simulink model "Attitude_control"  (R2021a)
settings: Solver=VariableStepAuto  StartTime=0.0  StopTime=200  RelTol=1e-3
values from neighbouring files (symbols this model uses):
  D = 9.4e-5*Kt    (= 4.7e-06)    [motor_parameter.m]
  Kt = 0.05    [motor_parameter.m]
  L = 0.001    [motor_parameter.m]
  R = 14.3    [motor_parameter.m]
undefined symbols (not defined in the file or in its folder): b, Is, Km, Q, q_init, Rgyro, Rstr, rw_Inertia, RW_Mmax, rw_SensorToBody, RW_wmax, Ts, unit7, w0, w_dot_init, w_init, wRW_init
libraries: pid_lib x11, simulink_extras x10, sharedtransform x5, simulink x3, aerolibutil x1, sharedTrackingLibrary x1
(part 1 of 2)
settings Model: Creator=sokserey  LastModifiedBy=sokserey

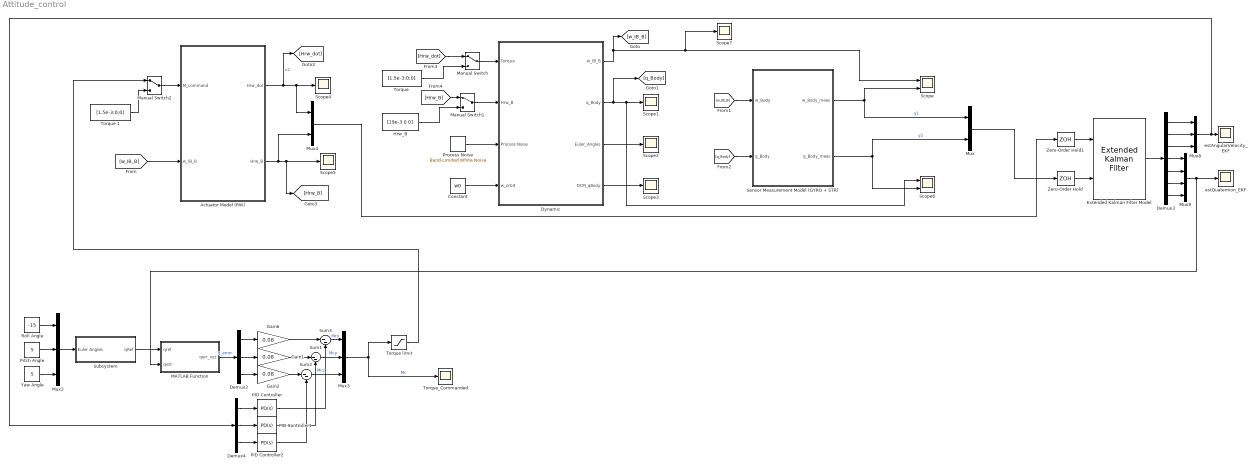
== system Attitude_control ==
  Actuator Model (RW) : Subsystem
  Constant : Constant  Value=w0
  Demux2 : Demux  Outputs=3
  Demux3 : Demux  Outputs=7
  Demux4 : Demux  Outputs=3
  Dynamic : Subsystem
  "Extended Kalman Filter Model " : sharedTrackingLibrary/Extended Kalman Filter  StateTransitionFcn=dynamicFunctions2  HasStateTransitionJacobianFcn=off  HasAdditiveProcessNoise=Additive  ProcessNoise=diag(unit7)*Q  HasTimeVaryingProcessNoise=off  HasStateTransitionFcnExtraArgument=1  InitialState=[w_init; q_init]  InitialStateCovariance=1e-6  MeasurementFcn1=measurementFunction2  HasMeasurementJacobianFcn1=off  HasMeasurementEnablePort1=off  HasAdditiveMeasurementNoise1=Additive  MeasurementNoise1=Rconf4  HasTimeVaryingMeasurementNoise1=off  HasMeasurementFcnExtraArgument1=0  MeasurementFcn2=myMeasurementFcn  HasMeasurementJacobianFcn2=off  HasMeasurementEnablePort2=off  HasAdditiveMeasurementNoise2=Additive  MeasurementNoise2=1  HasTimeVaryingMeasurementNoise2=off  HasMeasurementFcnExtraArgument2=0  MeasurementFcn3=myMeasurementFcn  HasMeasurementJacobianFcn3=off  HasMeasurementEnablePort3=off  HasAdditiveMeasurementNoise3=Additive  MeasurementNoise3=1  HasTimeVaryingMeasurementNoise3=off  HasMeasurementFcnExtraArgument3=0  MeasurementFcn4=myMeasurementFcn  HasMeasurementJacobianFcn4=off  HasMeasurementEnablePort4=off  HasAdditiveMeasurementNoise4=Additive  MeasurementNoise4=1  HasTimeVaryingMeasurementNoise4=off  HasMeasurementFcnExtraArgument4=0  MeasurementFcn5=myMeasurementFcn  HasMeasurementJacobianFcn5=off  HasMeasurementEnablePort5=off  HasAdditiveMeasurementNoise5=Additive  MeasurementNoise5=1  HasTimeVaryingMeasurementNoise5=off  HasMeasurementFcnExtraArgument5=0  EnableMultirate=off  StateTransitionFcnSampleTime=1  MeasurementFcn1SampleTime=1  MeasurementFcn2SampleTime=1  MeasurementFcn3SampleTime=1  MeasurementFcn4SampleTime=1  MeasurementFcn5SampleTime=1  UseCurrentEstimator=on  OutputStateCovariance=off  DataType=double  SampleTime=Ts  NumberOfMeasurements=1
      settings: SourceProductBaseCode=CT,DR,TF,ID,LP,NV,AR,RO,RR,UV,VE
  Gain1 : Gain  Gain=0.08
  Gain2 : Gain  Gain=0.08
  Gain6 : Gain  Gain=0.08
  Hrw_B : Constant  Value=[19e-3 0 0]
  MATLAB Function : MATLAB Function  TreatAsAtomicUnit=on
  Manual Switch : ManualSwitch
  Manual Switch1 : ManualSwitch
  Manual Switch2 : ManualSwitch
  Mux : Mux  Inputs=2
  Mux2 : Mux  Inputs=3
  Mux3 : Mux  Inputs=3
  Mux4 : Mux  Inputs=2
  Mux8 : Mux  Inputs=3
  Mux9 : Mux
  PID Controller : pid_lib/PID Controller  Controller=PD  Form=Parallel  TimeDomain=Continuous-time  UseExternalTs=off  SampleTime=-1  IntegratorMethod=Forward Euler  FilterMethod=Forward Euler  ControllerParametersSource=internal  P=1  I=2  D=2  UseFilter=on  N=100  TunerSelectOption=Transfer Function Based (PID Tuner App)  InitialConditionSource=internal  InitialConditionForIntegrator=0  InitialConditionForFilter=0  DifferentiatorICPrevScaledInput=0  ExternalReset=none  TrackingMode=off  Kt=1  LimitOutput=off  SatLimitsSource=internal  UpperSaturationLimit=inf  LowerSaturationLimit=-inf  LinearizeAsGain=on  AntiWindupMode=none  Kb=1  POutMin=[]  POutMax=[]  IOutMin=[]  IOutMax=[]  DOutMin=[]  DOutMax=[]  NOutMin=[]  NOutMax=[]  SumOutMin=[]  SumOutMax=[]  SaturationOutMin=[]  SaturationOutMax=[]  PParamMin=[]  PParamMax=[]  IParamMin=[]  IParamMax=[]  DParamMin=[]  DParamMax=[]  NParamMin=[]  NParamMax=[]  KbParamMin=[]  KbParamMax=[]  KtParamMin=[]  KtParamMax=[]  KbOutMin=[]  KbOutMax=[]  KtOutMin=[]  KtOutMax=[]  IntegratorOutMin=[]  IntegratorOutMax=[]  FilterOutMin=[]  FilterOutMax=[]  SumI1OutMin=[]  SumI1OutMax=[]  SumI2OutMin=[]  SumI2OutMax=[]  SumI3OutMin=[]  SumI3OutMax=[]  SumI4OutMin=[]  SumI4OutMax=[]  SumDOutMin=[]  SumDOutMax=[]  DifferentiatorOutMin=[]  DifferentiatorOutMax=[]  FilterDiffOutCoefMin=[]  FilterDiffOutCoefMax=[]  ReciprocalOutMin=[]  ReciprocalOutMax=[]  SumDenOutMin=[]  SumDenOutMax=[]  SumNumOutMin=[]  SumNumOutMax=[]  DivideOutMin=[]  DivideOutMax=[]  UdiffTsProdOutMin=[]  UdiffTsProdOutMax=[]  NTsProdOutMin=[]  NTsProdOutMax=[]  UintegralTsProdOutMin=[]  UintegralTsProdOutMax=[]  UngainTsProdOutMin=[]  UngainTsProdOutMax=[]  IntegratorContinuousStateAttributes=''  IntegratorStateMustResolveToSignalObject=off  IntegratorRTWStateStorageClass=Auto  FilterContinuousStateAttributes=''  FilterStateMustResolveToSignalObject=off  FilterRTWStateStorageClass=Auto  ParallelPVariant=InternalParameters  IdealPVariant=Disabled  IVariant=Disabled  DVariant=InternalParameters  IntegratorVariant=Disabled  SatVariant=Disabled  AWVariant=Disabled  PCopyVariant=Disabled  TRVariant=Disabled  FdbkBlocksVariant=Forward  IdealPFdbkVariant=Disabled  SatFdbkVariant=Disabled  DerivativeFilterVariant=ContFilter  NVariant=InternalParameters  NCopyVariant=Disabled  FilterICVariant=InternalICsFilter  IntegratorICVariant=Disabled  ExternalResetVariant=Disabled  TRSumVariant=Passthrough  SumFdbkVariant=Disabled  SumVariant=Sum_PD  TsampFilterVariant=InternalTs  TsampNgainVariant=Passthrough  TsampIntegralVariant=Disabled_SignalSpec  ExternalSaturationOutDataTypeStr=Inherit: Same as second input
  PID Controller1 : pid_lib/PID Controller  Controller=PD  Form=Parallel  TimeDomain=Continuous-time  UseExternalTs=off  SampleTime=-1  IntegratorMethod=Forward Euler  FilterMethod=Forward Euler  ControllerParametersSource=internal  P=1  I=2  D=2  UseFilter=on  N=100  TunerSelectOption=Transfer Function Based (PID Tuner App)  InitialConditionSource=internal  InitialConditionForIntegrator=0  InitialConditionForFilter=0  DifferentiatorICPrevScaledInput=0  ExternalReset=none  TrackingMode=off  Kt=1  LimitOutput=off  SatLimitsSource=internal  UpperSaturationLimit=inf  LowerSaturationLimit=-inf  LinearizeAsGain=on  AntiWindupMode=none  Kb=1  POutMin=[]  POutMax=[]  IOutMin=[]  IOutMax=[]  DOutMin=[]  DOutMax=[]  NOutMin=[]  NOutMax=[]  SumOutMin=[]  SumOutMax=[]  SaturationOutMin=[]  SaturationOutMax=[]  PParamMin=[]  PParamMax=[]  IParamMin=[]  IParamMax=[]  DParamMin=[]  DParamMax=[]  NParamMin=[]  NParamMax=[]  KbParamMin=[]  KbParamMax=[]  KtParamMin=[]  KtParamMax=[]  KbOutMin=[]  KbOutMax=[]  KtOutMin=[]  KtOutMax=[]  IntegratorOutMin=[]  IntegratorOutMax=[]  FilterOutMin=[]  FilterOutMax=[]  SumI1OutMin=[]  SumI1OutMax=[]  SumI2OutMin=[]  SumI2OutMax=[]  SumI3OutMin=[]  SumI3OutMax=[]  SumI4OutMin=[]  SumI4OutMax=[]  SumDOutMin=[]  SumDOutMax=[]  DifferentiatorOutMin=[]  DifferentiatorOutMax=[]  FilterDiffOutCoefMin=[]  FilterDiffOutCoefMax=[]  ReciprocalOutMin=[]  ReciprocalOutMax=[]  SumDenOutMin=[]  SumDenOutMax=[]  SumNumOutMin=[]  SumNumOutMax=[]  DivideOutMin=[]  DivideOutMax=[]  UdiffTsProdOutMin=[]  UdiffTsProdOutMax=[]  NTsProdOutMin=[]  NTsProdOutMax=[]  UintegralTsProdOutMin=[]  UintegralTsProdOutMax=[]  UngainTsProdOutMin=[]  UngainTsProdOutMax=[]  IntegratorContinuousStateAttributes=''  IntegratorStateMustResolveToSignalObject=off  IntegratorRTWStateStorageClass=Auto  FilterContinuousStateAttributes=''  FilterStateMustResolveToSignalObject=off  FilterRTWStateStorageClass=Auto  ParallelPVariant=InternalParameters  IdealPVariant=Disabled  IVariant=Disabled  DVariant=InternalParameters  IntegratorVariant=Disabled  SatVariant=Disabled  AWVariant=Disabled  PCopyVariant=Disabled  TRVariant=Disabled  FdbkBlocksVariant=Forward  IdealPFdbkVariant=Disabled  SatFdbkVariant=Disabled  DerivativeFilterVariant=ContFilter  NVariant=InternalParameters  NCopyVariant=Disabled  FilterICVariant=InternalICsFilter  IntegratorICVariant=Disabled  ExternalResetVariant=Disabled  TRSumVariant=Passthrough  SumFdbkVariant=Disabled  SumVariant=Sum_PD  TsampFilterVariant=InternalTs  TsampNgainVariant=Passthrough  TsampIntegralVariant=Disabled_SignalSpec  ExternalSaturationOutDataTypeStr=Inherit: Same as second input
  PID Controller2 : pid_lib/PID Controller  Controller=PD  Form=Parallel  TimeDomain=Continuous-time  UseExternalTs=off  SampleTime=-1  IntegratorMethod=Forward Euler  FilterMethod=Forward Euler  ControllerParametersSource=internal  P=1  I=2  D=2  UseFilter=on  N=100  TunerSelectOption=Transfer Function Based (PID Tuner App)  InitialConditionSource=internal  InitialConditionForIntegrator=0  InitialConditionForFilter=0  DifferentiatorICPrevScaledInput=0  ExternalReset=none  TrackingMode=off  Kt=1  LimitOutput=off  SatLimitsSource=internal  UpperSaturationLimit=inf  LowerSaturationLimit=-inf  LinearizeAsGain=on  AntiWindupMode=none  Kb=1  POutMin=[]  POutMax=[]  IOutMin=[]  IOutMax=[]  DOutMin=[]  DOutMax=[]  NOutMin=[]  NOutMax=[]  SumOutMin=[]  SumOutMax=[]  SaturationOutMin=[]  SaturationOutMax=[]  PParamMin=[]  PParamMax=[]  IParamMin=[]  IParamMax=[]  DParamMin=[]  DParamMax=[]  NParamMin=[]  NParamMax=[]  KbParamMin=[]  KbParamMax=[]  KtParamMin=[]  KtParamMax=[]  KbOutMin=[]  KbOutMax=[]  KtOutMin=[]  KtOutMax=[]  IntegratorOutMin=[]  IntegratorOutMax=[]  FilterOutMin=[]  FilterOutMax=[]  SumI1OutMin=[]  SumI1OutMax=[]  SumI2OutMin=[]  SumI2OutMax=[]  SumI3OutMin=[]  SumI3OutMax=[]  SumI4OutMin=[]  SumI4OutMax=[]  SumDOutMin=[]  SumDOutMax=[]  DifferentiatorOutMin=[]  DifferentiatorOutMax=[]  FilterDiffOutCoefMin=[]  FilterDiffOutCoefMax=[]  ReciprocalOutMin=[]  ReciprocalOutMax=[]  SumDenOutMin=[]  SumDenOutMax=[]  SumNumOutMin=[]  SumNumOutMax=[]  DivideOutMin=[]  DivideOutMax=[]  UdiffTsProdOutMin=[]  UdiffTsProdOutMax=[]  NTsProdOutMin=[]  NTsProdOutMax=[]  UintegralTsProdOutMin=[]  UintegralTsProdOutMax=[]  UngainTsProdOutMin=[]  UngainTsProdOutMax=[]  IntegratorContinuousStateAttributes=''  IntegratorStateMustResolveToSignalObject=off  IntegratorRTWStateStorageClass=Auto  FilterContinuousStateAttributes=''  FilterStateMustResolveToSignalObject=off  FilterRTWStateStorageClass=Auto  ParallelPVariant=InternalParameters  IdealPVariant=Disabled  IVariant=Disabled  DVariant=InternalParameters  IntegratorVariant=Disabled  SatVariant=Disabled  AWVariant=Disabled  PCopyVariant=Disabled  TRVariant=Disabled  FdbkBlocksVariant=Forward  IdealPFdbkVariant=Disabled  SatFdbkVariant=Disabled  DerivativeFilterVariant=ContFilter  NVariant=InternalParameters  NCopyVariant=Disabled  FilterICVariant=InternalICsFilter  IntegratorICVariant=Disabled  ExternalResetVariant=Disabled  TRSumVariant=Passthrough  SumFdbkVariant=Disabled  SumVariant=Sum_PD  TsampFilterVariant=InternalTs  TsampNgainVariant=Passthrough  TsampIntegralVariant=Disabled_SignalSpec  ExternalSaturationOutDataTypeStr=Inherit: Same as second input
  Pitch Angle : Constant  Value=5
  Process Noise : simulink/Sources/Band-Limited White Noise  Cov=Q*Ts  Ts=Ts  seed=[23341]
  Roll Angle : Constant  Value=-15
  Scope : Scope  NumInputPorts=2
  Scope{1..5,7} (6 alike) : Scope
  Scope6 : Scope  NumInputPorts=2
  Sensor Measurement Model (GYRO + STR) : Subsystem
  Subsystem : Subsystem
  Sum1 : Sum  Inputs=|--
  Sum2 : Sum  Inputs=|--
  Sum3 : Sum  Inputs=|--
  Torque limit : Saturate  UpperLimit=RW_Mmax  LowerLimit=-RW_Mmax
  "Torque " : Constant  Value=[1.5e-3;0;0]
  Torque 1 : Constant  Value=[1.5e-3;0;0]
  Torque_Commanded : Scope
  Yaw Angle : Constant  Value=5
  Zero-Order Hold : ZeroOrderHold  SampleTime=Ts
  Zero-Order Hold1 : ZeroOrderHold  SampleTime=Ts
  estAngularVelocity_EKF : Scope
  "estQuaternion_EKF " : Scope
  wires:
  Process Noise/1 -> Dynamic/3("Process Noise ")
  Constant/1 -> Dynamic/4(w_orbit)
  Dynamic/1(w_IB_B) -> [w_IB_B], Scope7/1, Scope/1
  Dynamic/2(q_Body) -> [q_Body], Scope6/1, Scope1/1
  Dynamic/3(Euler_Angles) -> Scope2/1
  Dynamic/4(DCM_qBody) -> Scope3/1
  Zero-Order Hold1/1 -> "Extended Kalman Filter Model "/1
  Demux3/2 -> Mux8/2
  Demux3/3 -> Mux8/3
  Demux3/6 -> Mux9/3
  Demux3/4 -> Mux9/1
  Mux9/1 -> "estQuaternion_EKF "/1, MATLAB Function/2(qest)
  Demux3/5 -> Mux9/2
  "Extended Kalman Filter Model "/1 -> Demux3/1
  Demux3/1 -> Mux8/1
  Zero-Order Hold/1 -> "Extended Kalman Filter Model "/2
  [w_IB_B] -> Actuator Model (RW)/2(w_IB_B)
  Actuator Model (RW)/1("Hrw_dot ") -> [Hrw_dot], Mux4/1, Scope4/1  "u1"
  Actuator Model (RW)/2(Hrw_B) -> Mux4/2, [Hrw_B], Scope5/1
  [w_IB_B] -> Sensor Measurement Model (GYRO + STR)/1(w_Body)
  Sensor Measurement Model (GYRO + STR)/1(w_Body_meas) -> Mux/1, Scope/2  "y1"
  [q_Body] -> Sensor Measurement Model (GYRO + STR)/2(q_Body)
  Sensor Measurement Model (GYRO + STR)/2(q_Body_meas) -> Mux/2, Scope6/2  "y2"
  Mux/1 -> Zero-Order Hold/1
  Manual Switch/1 -> Dynamic/1(Torque)
  "Torque "/1 -> Manual Switch/2
  Manual Switch1/1 -> Dynamic/2(Hrw_B)
  Hrw_B/1 -> Manual Switch1/2
  [Hrw_dot] -> Manual Switch/1
  [Hrw_B] -> Manual Switch1/1
  Roll Angle/1 -> Mux2/1
  Sum1/1 -> Mux3/2  "Mcy"
  MATLAB Function/1(qerr_xyz) -> Demux2/1  "q_error"
  Demux4/2 -> PID Controller1/1
  PID Controller2/1 -> Sum2/2
  Sum3/1 -> Mux3/1  "Mcx"
  Gain2/1 -> Sum2/1
  PID Controller/1 -> Sum3/2
  PID Controller1/1 -> Sum1/2
  Sum2/1 -> Mux3/3  "Mcz"
  Demux4/1 -> PID Controller/1
  Demux2/2 -> Gain1/1
  Demux2/1 -> Gain6/1
  Gain6/1 -> Sum3/1
  Mux3/1 -> Torque limit/1, Torque_Commanded/1  "Mc"
  Yaw Angle/1 -> Mux2/3
  Subsystem/1(qRef) -> MATLAB Function/1(qref)
  Gain1/1 -> Sum1/1
  Pitch Angle/1 -> Mux2/2
  Mux2/1 -> Subsystem/1(Euler Angles)
  Demux2/3 -> Gain2/1
  Mux8/1 -> Demux4/1, estAngularVelocity_EKF/1
  Demux4/3 -> PID Controller2/1
  Torque limit/1 -> Manual Switch2/1
  Manual Switch2/1 -> Actuator Model (RW)/1("M_command ")
  Torque 1/1 -> Manual Switch2/2
  Demux3/7 -> Mux9/4
  Mux4/1 -> Zero-Order Hold1/1

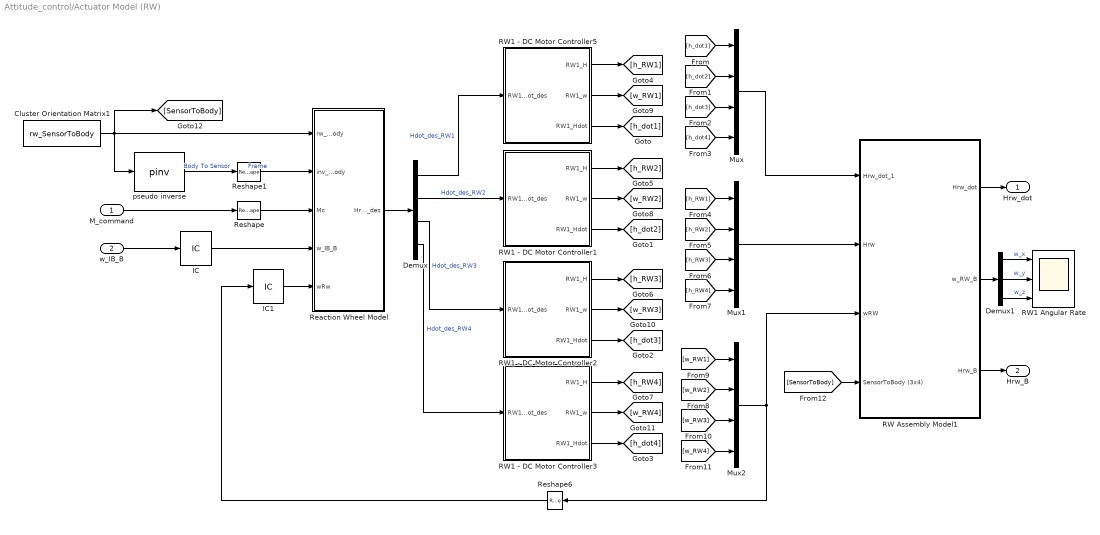
== system Attitude_control/Actuator Model (RW) ==
  "M_command " : Inport
  w_IB_B : Inport  Port=2
  Cluster Orientation Matrix1 : Constant  Value=rw_SensorToBody  VectorParams1D=off  SampleTime=Ts
  Demux : Demux
  Demux1 : Demux  Outputs=3
  IC : InitialCondition  Value=w_init
  IC1 : InitialCondition  Value=wRW_init
  Mux : Mux
  Mux1 : Mux
  Mux2 : Mux
  RW Assembly Model1 : Subsystem
  RW1 - DC Motor Controller1 : Subsystem
  RW1 - DC Motor Controller2 : Subsystem
  RW1 - DC Motor Controller3 : Subsystem
  RW1 - DC Motor Controller5 : Subsystem
  RW1 Angular Rate : Scope  NumInputPorts=3
  Reaction Wheel Model : MATLAB Function  TreatAsAtomicUnit=on
  Reshape : Reshape  OutputDimensionality=Column vector (2-D)
  Reshape1 : Reshape  OutputDimensionality=Customize  OutputDimensions=[4,3]
  Reshape6 : Reshape  OutputDimensionality=Column vector (2-D)
  pseudo inverse : MATLABFcn  MATLABFcn=pinv
  "Hrw_dot " : Outport  VectorParamsAs1DForOutWhenUnconnected=off
  Hrw_B : Outport  Port=2  VectorParamsAs1DForOutWhenUnconnected=off
  wires:
  Demux/1 -> RW1 - DC Motor Controller5/1(RW1_Hdot_des)  "Hdot_des_RW1"
  Demux/2 -> RW1 - DC Motor Controller1/1(RW1_Hdot_des)  "Hdot_des_RW2"
  Demux/3 -> RW1 - DC Motor Controller2/1(RW1_Hdot_des)  "Hdot_des_RW3"
  Demux/4 -> RW1 - DC Motor Controller3/1(RW1_Hdot_des)  "Hdot_des_RW4"
  Demux1/3 -> RW1 Angular Rate/3  "w_z"
  Demux1/1 -> RW1 Angular Rate/1  "w_x"
  Demux1/2 -> RW1 Angular Rate/2  "w_y"
  "M_command "/1 -> Reshape/1
  Reaction Wheel Model/1(Hrw_dot_des) -> Demux/1
  [h_dot1] -> Mux/1
  [h_dot2] -> Mux/2
  [h_dot3] -> Mux/3
  [h_dot4] -> Mux/4
  Mux/1 -> RW Assembly Model1/1(Hrw_dot_1)
  [h_RW1] -> Mux1/1
  [h_RW2] -> Mux1/2
  [h_RW3] -> Mux1/3
  [h_RW4] -> Mux1/4
  Mux1/1 -> RW Assembly Model1/2(Hrw)
  [w_RW2] -> Mux2/2
  [w_RW1] -> Mux2/1
  [w_RW3] -> Mux2/3
  [w_RW4] -> Mux2/4
  pseudo inverse/1 -> Reshape1/1  "Body To Sensor         Frame"
  Reshape/1 -> Reaction Wheel Model/3(Mc)
  Cluster Orientation Matrix1/1 -> pseudo inverse/1, [SensorToBody], Reaction Wheel Model/1(rw_SensorToBody)
  [SensorToBody] -> RW Assembly Model1/4(SensorToBody (3x4))
  RW Assembly Model1/2(w_RW_B) -> Demux1/1
  RW Assembly Model1/1(Hrw_dot) -> "Hrw_dot "/1
  Mux2/1 -> Reshape6/1, RW Assembly Model1/3(wRW)
  Reshape6/1 -> IC1/1
  Reshape1/1 -> Reaction Wheel Model/2(inv_rwSensorToBody)
  w_IB_B/1 -> IC/1
  IC/1 -> Reaction Wheel Model/4(w_IB_B)
  IC1/1 -> Reaction Wheel Model/5(wRw)
  RW1 - DC Motor Controller5/2(RW1_w) -> [w_RW1]
  RW1 - DC Motor Controller5/1(RW1_H) -> [h_RW1]
  RW1 - DC Motor Controller5/3(RW1_Hdot) -> [h_dot1]
  RW1 - DC Motor Controller1/1(RW1_H) -> [h_RW2]
  RW1 - DC Motor Controller1/2(RW1_w) -> [w_RW2]
  RW1 - DC Motor Controller1/3(RW1_Hdot) -> [h_dot2]
  RW1 - DC Motor Controller2/1(RW1_H) -> [h_RW3]
  RW1 - DC Motor Controller2/2(RW1_w) -> [w_RW3]
  RW1 - DC Motor Controller2/3(RW1_Hdot) -> [h_dot3]
  RW1 - DC Motor Controller3/1(RW1_H) -> [h_RW4]
  RW1 - DC Motor Controller3/2(RW1_w) -> [w_RW4]
  RW1 - DC Motor Controller3/3(RW1_Hdot) -> [h_dot4]
  RW Assembly Model1/3(Hrw_B) -> Hrw_B/1

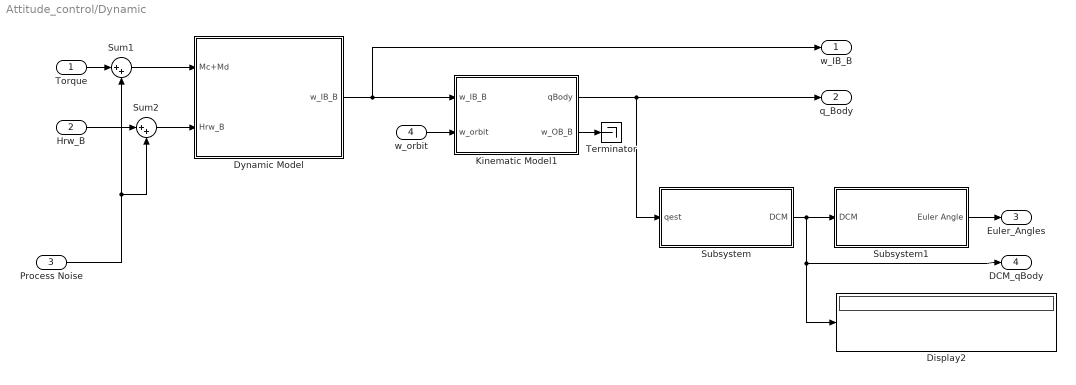
== system Attitude_control/Dynamic ==
  Torque : Inport
  Hrw_B : Inport  Port=2
  "Process Noise " : Inport  Port=3
  w_orbit : Inport  Port=4
  Display2 : Display
  Dynamic Model : Subsystem
  Kinematic Model1 : Subsystem
  Subsystem : Subsystem
  Subsystem1 : Subsystem
  Sum1 : Sum  Inputs=|++
  Sum2 : Sum  Inputs=|++
  Terminator : Terminator
  w_IB_B : Outport  VectorParamsAs1DForOutWhenUnconnected=off
  q_Body : Outport  Port=2  VectorParamsAs1DForOutWhenUnconnected=off
  Euler_Angles : Outport  Port=3  VectorParamsAs1DForOutWhenUnconnected=off
  DCM_qBody : Outport  Port=4  VectorParamsAs1DForOutWhenUnconnected=off
  wires:
  Sum2/1 -> Dynamic Model/2("Hrw_B ")
  Dynamic Model/1(w_IB_B) -> Kinematic Model1/1(w_IB_B), w_IB_B/1
  Hrw_B/1 -> Sum2/1
  Sum1/1 -> Dynamic Model/1(Mc+Md)
  Subsystem1/1(Euler Angle) -> Euler_Angles/1
  Torque/1 -> Sum1/1
  Kinematic Model1/2(w_OB_B) -> Terminator/1
  Kinematic Model1/1(qBody) -> Subsystem/1(qest), q_Body/1
  "Process Noise "/1 -> Sum2/2, Sum1/2
  Subsystem/1("DCM ") -> Display2/1, DCM_qBody/1, Subsystem1/1("DCM ")
  w_orbit/1 -> Kinematic Model1/2(w_orbit)

== system Attitude_control/Sensor Measurement Model (GYRO + STR) ==
  w_Body : Inport
  q_Body : Inport  Port=2
  GYRO Sensor Model : Subsystem
  Normalization Model : Subsystem
  Star Tracker Model : Subsystem
  w_Body_meas : Outport  VectorParamsAs1DForOutWhenUnconnected=off
  q_Body_meas : Outport  Port=2  VectorParamsAs1DForOutWhenUnconnected=off
  wires:
  GYRO Sensor Model/1(w_Body_meas) -> w_Body_meas/1
  w_Body/1 -> GYRO Sensor Model/1(w_Body)
  q_Body/1 -> Star Tracker Model/1(q_Body)
  Normalization Model/1(Normalized_u) -> q_Body_meas/1
  Star Tracker Model/1(q_Body_meas) -> Normalization Model/1(u)

== system Attitude_control/Subsystem ==
  Euler Angles : Inport
  Degrees to Radians1 : simulink_extras/Transformations/Degrees to Radians
  Direction Cosine Matrix to Quaternions : sharedtransform/Direction Cosine Matrix  to Quaternions  aMode=0  action=None  tolerance=eps(2)
      settings: SourceProductBaseCode=AE,PW,DR,MT,UV,VE
  Rotation Angles to Direction Cosine Matrix : sharedtransform/Rotation Angles to Direction Cosine Matrix  rotationOrder=ZYX  aMode=aMode
      settings: SourceProductBaseCode=AE,PW,DR,MT,UV,VE
  Subsystem1 : Subsystem
  qRef : Outport  VectorParamsAs1DForOutWhenUnconnected=off
  wires:
  Euler Angles/1 -> Degrees to Radians1/1
  Degrees to Radians1/1 -> Rotation Angles to Direction Cosine Matrix/1
  Rotation Angles to Direction Cosine Matrix/1 -> Direction Cosine Matrix to Quaternions/1
  Direction Cosine Matrix to Quaternions/1 -> Subsystem1/1(q0,q1,q2,q3)
  Subsystem1/1(q1,q2,q3,q4) -> qRef/1

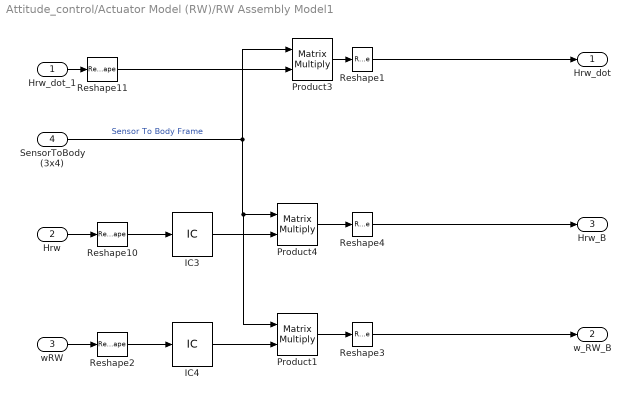
== system Attitude_control/Actuator Model (RW)/RW Assembly Model1 ==
  Hrw_dot_1 : Inport
  Hrw : Inport  Port=2
  wRW : Inport  Port=3
  SensorToBody (3x4) : Inport  Port=4
  IC3 : InitialCondition  Value=[wRW_init(1,1)*rw_Inertia; wRW_init(2,1)*rw_Inertia; wRW_init(3,1)*rw_Inertia;wRW_init(4,1)*rw_Inertia]
  IC4 : InitialCondition  Value=wRW_init
  Product1 : Product  Inputs=**  Multiplication=Matrix(*)  RndMeth=Zero
  Product3 : Product  Inputs=**  Multiplication=Matrix(*)  RndMeth=Zero
  Product4 : Product  Inputs=**  Multiplication=Matrix(*)  RndMeth=Zero
  Reshape{1..4,10..11} (6 alike) : Reshape  OutputDimensionality=Column vector (2-D)
  Hrw_dot : Outport  VectorParamsAs1DForOutWhenUnconnected=off
  w_RW_B : Outport  Port=2  VectorParamsAs1DForOutWhenUnconnected=off
  Hrw_B : Outport  Port=3  VectorParamsAs1DForOutWhenUnconnected=off
  wires:
  SensorToBody (3x4)/1 -> Product3/1, Product1/1, Product4/1  "Sensor To Body Frame"
  Product4/1 -> Reshape4/1
  Reshape1/1 -> Hrw_dot/1
  Reshape4/1 -> Hrw_B/1
  IC3/1 -> Product4/2
  IC4/1 -> Product1/2
  Product1/1 -> Reshape3/1
  Hrw/1 -> Reshape10/1
  Reshape10/1 -> IC3/1
  Reshape2/1 -> IC4/1
  wRW/1 -> Reshape2/1
  Reshape3/1 -> w_RW_B/1
  Reshape11/1 -> Product3/2
  Hrw_dot_1/1 -> Reshape11/1
  Product3/1 -> Reshape1/1

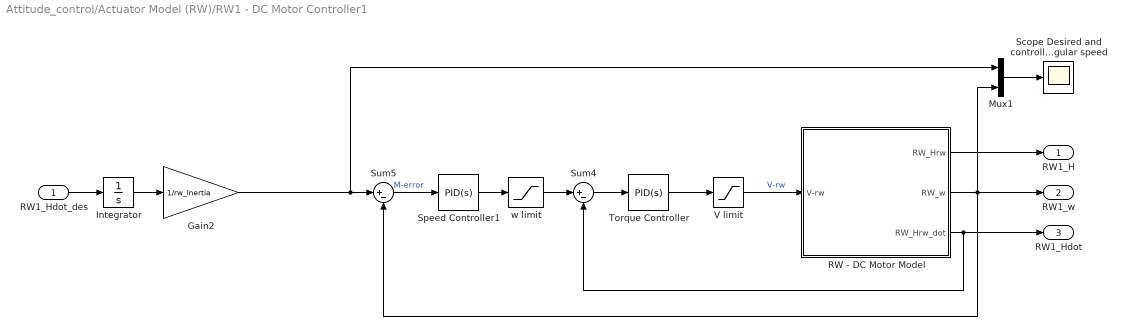
== system Attitude_control/Actuator Model (RW)/RW1 - DC Motor Controller1 ==
  RW1_Hdot_des : Inport
  Gain2 : Gain  Gain=1/rw_Inertia
  Integrator : Integrator
  Mux1 : Mux  Inputs=2
  RW - DC Motor Model : Subsystem
  "Scope Desired and controlled RW-angular speed " : Scope
  Speed Controller1 : pid_lib/PID Controller  Controller=PID  Form=Parallel  TimeDomain=Continuous-time  UseExternalTs=off  SampleTime=0.01  IntegratorMethod=Forward Euler  FilterMethod=Forward Euler  ControllerParametersSource=internal  P=9.56052273582853  I=13.4366327144231  D=1.16248121318414  UseFilter=on  N=2668.95305381072  TunerSelectOption=Transfer Function Based (PID Tuner App)  InitialConditionSource=internal  InitialConditionForIntegrator=0  InitialConditionForFilter=0  DifferentiatorICPrevScaledInput=0  ExternalReset=none  TrackingMode=off  Kt=1  LimitOutput=off  SatLimitsSource=internal  UpperSaturationLimit=inf  LowerSaturationLimit=-inf  LinearizeAsGain=on  AntiWindupMode=none  Kb=1  POutMin=[]  POutMax=[]  IOutMin=[]  IOutMax=[]  DOutMin=[]  DOutMax=[]  NOutMin=[]  NOutMax=[]  SumOutMin=[]  SumOutMax=[]  SaturationOutMin=[]  SaturationOutMax=[]  PParamMin=[]  PParamMax=[]  IParamMin=[]  IParamMax=[]  DParamMin=[]  DParamMax=[]  NParamMin=[]  NParamMax=[]  KbParamMin=[]  KbParamMax=[]  KtParamMin=[]  KtParamMax=[]  KbOutMin=[]  KbOutMax=[]  KtOutMin=[]  KtOutMax=[]  IntegratorOutMin=[]  IntegratorOutMax=[]  FilterOutMin=[]  FilterOutMax=[]  SumI1OutMin=[]  SumI1OutMax=[]  SumI2OutMin=[]  SumI2OutMax=[]  SumI3OutMin=[]  SumI3OutMax=[]  SumI4OutMin=[]  SumI4OutMax=[]  SumDOutMin=[]  SumDOutMax=[]  DifferentiatorOutMin=[]  DifferentiatorOutMax=[]  FilterDiffOutCoefMin=[]  FilterDiffOutCoefMax=[]  ReciprocalOutMin=[]  ReciprocalOutMax=[]  SumDenOutMin=[]  SumDenOutMax=[]  SumNumOutMin=[]  SumNumOutMax=[]  DivideOutMin=[]  DivideOutMax=[]  UdiffTsProdOutMin=[]  UdiffTsProdOutMax=[]  NTsProdOutMin=[]  NTsProdOutMax=[]  UintegralTsProdOutMin=[]  UintegralTsProdOutMax=[]  UngainTsProdOutMin=[]  UngainTsProdOutMax=[]  IntegratorContinuousStateAttributes=''  IntegratorStateMustResolveToSignalObject=off  IntegratorRTWStateStorageClass=Auto  FilterContinuousStateAttributes=''  FilterStateMustResolveToSignalObject=off  FilterRTWStateStorageClass=Auto  ParallelPVariant=InternalParameters  IdealPVariant=Disabled  IVariant=InternalParameters  DVariant=InternalParameters  IntegratorVariant=Continuous  SatVariant=Disabled  AWVariant=Passthrough  PCopyVariant=Disabled  TRVariant=Disabled  FdbkBlocksVariant=Forward  IdealPFdbkVariant=Disabled  SatFdbkVariant=Disabled  DerivativeFilterVariant=ContFilter  NVariant=InternalParameters  NCopyVariant=Disabled  FilterICVariant=InternalICsFilter  IntegratorICVariant=InternalICs  ExternalResetVariant=Disabled  TRSumVariant=Passthrough  SumFdbkVariant=Disabled  SumVariant=Sum_PID  TsampFilterVariant=InternalTs  TsampNgainVariant=Passthrough  TsampIntegralVariant=Passthrough  ExternalSaturationOutDataTypeStr=Inherit: Same as second input
  Sum4 : Sum  Inputs=|+-
  Sum5 : Sum  Inputs=|+-
  Torque Controller : pid_lib/PID Controller  Controller=PID  Form=Parallel  TimeDomain=Continuous-time  UseExternalTs=off  SampleTime=0.01  IntegratorMethod=Forward Euler  FilterMethod=Forward Euler  ControllerParametersSource=internal  P=2.50374683332827e-05  I=0.022215359014968  D=0  UseFilter=on  N=100  TunerSelectOption=Transfer Function Based (PID Tuner App)  InitialConditionSource=internal  InitialConditionForIntegrator=0  InitialConditionForFilter=0  DifferentiatorICPrevScaledInput=0  ExternalReset=none  TrackingMode=off  Kt=1  LimitOutput=off  SatLimitsSource=internal  UpperSaturationLimit=inf  LowerSaturationLimit=-inf  LinearizeAsGain=on  AntiWindupMode=none  Kb=1  POutMin=[]  POutMax=[]  IOutMin=[]  IOutMax=[]  DOutMin=[]  DOutMax=[]  NOutMin=[]  NOutMax=[]  SumOutMin=[]  SumOutMax=[]  SaturationOutMin=[]  SaturationOutMax=[]  PParamMin=[]  PParamMax=[]  IParamMin=[]  IParamMax=[]  DParamMin=[]  DParamMax=[]  NParamMin=[]  NParamMax=[]  KbParamMin=[]  KbParamMax=[]  KtParamMin=[]  KtParamMax=[]  KbOutMin=[]  KbOutMax=[]  KtOutMin=[]  KtOutMax=[]  IntegratorOutMin=[]  IntegratorOutMax=[]  FilterOutMin=[]  FilterOutMax=[]  SumI1OutMin=[]  SumI1OutMax=[]  SumI2OutMin=[]  SumI2OutMax=[]  SumI3OutMin=[]  SumI3OutMax=[]  SumI4OutMin=[]  SumI4OutMax=[]  SumDOutMin=[]  SumDOutMax=[]  DifferentiatorOutMin=[]  DifferentiatorOutMax=[]  FilterDiffOutCoefMin=[]  FilterDiffOutCoefMax=[]  ReciprocalOutMin=[]  ReciprocalOutMax=[]  SumDenOutMin=[]  SumDenOutMax=[]  SumNumOutMin=[]  SumNumOutMax=[]  DivideOutMin=[]  DivideOutMax=[]  UdiffTsProdOutMin=[]  UdiffTsProdOutMax=[]  NTsProdOutMin=[]  NTsProdOutMax=[]  UintegralTsProdOutMin=[]  UintegralTsProdOutMax=[]  UngainTsProdOutMin=[]  UngainTsProdOutMax=[]  IntegratorContinuousStateAttributes=''  IntegratorStateMustResolveToSignalObject=off  IntegratorRTWStateStorageClass=Auto  FilterContinuousStateAttributes=''  FilterStateMustResolveToSignalObject=off  FilterRTWStateStorageClass=Auto  ParallelPVariant=InternalParameters  IdealPVariant=Disabled  IVariant=InternalParameters  DVariant=InternalParameters  IntegratorVariant=Continuous  SatVariant=Disabled  AWVariant=Passthrough  PCopyVariant=Disabled  TRVariant=Disabled  FdbkBlocksVariant=Forward  IdealPFdbkVariant=Disabled  SatFdbkVariant=Disabled  DerivativeFilterVariant=ContFilter  NVariant=InternalParameters  NCopyVariant=Disabled  FilterICVariant=InternalICsFilter  IntegratorICVariant=InternalICs  ExternalResetVariant=Disabled  TRSumVariant=Passthrough  SumFdbkVariant=Disabled  SumVariant=Sum_PID  TsampFilterVariant=InternalTs  TsampNgainVariant=Passthrough  TsampIntegralVariant=Passthrough  ExternalSaturationOutDataTypeStr=Inherit: Same as second input
  V limit : Saturate  UpperLimit=20  LowerLimit=-20
  w limit : Saturate  UpperLimit=RW_wmax  LowerLimit=-RW_wmax
  RW1_H : Outport  VectorParamsAs1DForOutWhenUnconnected=off
  RW1_w : Outport  Port=2  VectorParamsAs1DForOutWhenUnconnected=off
  RW1_Hdot : Outport  Port=3  VectorParamsAs1DForOutWhenUnconnected=off
  wires:
  Integrator/1 -> Gain2/1
  RW1_Hdot_des/1 -> Integrator/1
  Mux1/1 -> "Scope Desired and controlled RW-angular speed "/1
  Sum5/1 -> Speed Controller1/1  "M-error"
  RW - DC Motor Model/3(RW_Hrw_dot) -> RW1_Hdot/1, Sum4/2
  Torque Controller/1 -> V limit/1
  Speed Controller1/1 -> w limit/1
  Gain2/1 -> Mux1/1, Sum5/1
  RW - DC Motor Model/2(RW_w) -> RW1_w/1, Sum5/2, Mux1/2
  Sum4/1 -> Torque Controller/1
  w limit/1 -> Sum4/1
  V limit/1 -> RW - DC Motor Model/1(V-rw)  "V-rw"
  RW - DC Motor Model/1(RW_Hrw) -> RW1_H/1

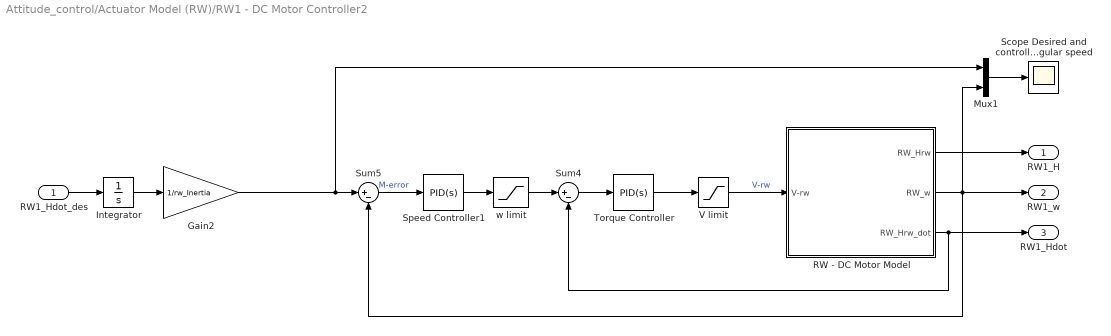
== system Attitude_control/Actuator Model (RW)/RW1 - DC Motor Controller2 ==
  RW1_Hdot_des : Inport
  Gain2 : Gain  Gain=1/rw_Inertia
  Integrator : Integrator
  Mux1 : Mux  Inputs=2
  RW - DC Motor Model : Subsystem
  "Scope Desired and controlled RW-angular speed " : Scope
  Speed Controller1 : pid_lib/PID Controller  Controller=PID  Form=Parallel  TimeDomain=Continuous-time  UseExternalTs=off  SampleTime=0.01  IntegratorMethod=Forward Euler  FilterMethod=Forward Euler  ControllerParametersSource=internal  P=9.56052273582853  I=13.4366327144231  D=1.16248121318414  UseFilter=on  N=2668.95305381072  TunerSelectOption=Transfer Function Based (PID Tuner App)  InitialConditionSource=internal  InitialConditionForIntegrator=0  InitialConditionForFilter=0  DifferentiatorICPrevScaledInput=0  ExternalReset=none  TrackingMode=off  Kt=1  LimitOutput=off  SatLimitsSource=internal  UpperSaturationLimit=inf  LowerSaturationLimit=-inf  LinearizeAsGain=on  AntiWindupMode=none  Kb=1  POutMin=[]  POutMax=[]  IOutMin=[]  IOutMax=[]  DOutMin=[]  DOutMax=[]  NOutMin=[]  NOutMax=[]  SumOutMin=[]  SumOutMax=[]  SaturationOutMin=[]  SaturationOutMax=[]  PParamMin=[]  PParamMax=[]  IParamMin=[]  IParamMax=[]  DParamMin=[]  DParamMax=[]  NParamMin=[]  NParamMax=[]  KbParamMin=[]  KbParamMax=[]  KtParamMin=[]  KtParamMax=[]  KbOutMin=[]  KbOutMax=[]  KtOutMin=[]  KtOutMax=[]  IntegratorOutMin=[]  IntegratorOutMax=[]  FilterOutMin=[]  FilterOutMax=[]  SumI1OutMin=[]  SumI1OutMax=[]  SumI2OutMin=[]  SumI2OutMax=[]  SumI3OutMin=[]  SumI3OutMax=[]  SumI4OutMin=[]  SumI4OutMax=[]  SumDOutMin=[]  SumDOutMax=[]  DifferentiatorOutMin=[]  DifferentiatorOutMax=[]  FilterDiffOutCoefMin=[]  FilterDiffOutCoefMax=[]  ReciprocalOutMin=[]  ReciprocalOutMax=[]  SumDenOutMin=[]  SumDenOutMax=[]  SumNumOutMin=[]  SumNumOutMax=[]  DivideOutMin=[]  DivideOutMax=[]  UdiffTsProdOutMin=[]  UdiffTsProdOutMax=[]  NTsProdOutMin=[]  NTsProdOutMax=[]  UintegralTsProdOutMin=[]  UintegralTsProdOutMax=[]  UngainTsProdOutMin=[]  UngainTsProdOutMax=[]  IntegratorContinuousStateAttributes=''  IntegratorStateMustResolveToSignalObject=off  IntegratorRTWStateStorageClass=Auto  FilterContinuousStateAttributes=''  FilterStateMustResolveToSignalObject=off  FilterRTWStateStorageClass=Auto  ParallelPVariant=InternalParameters  IdealPVariant=Disabled  IVariant=InternalParameters  DVariant=InternalParameters  IntegratorVariant=Continuous  SatVariant=Disabled  AWVariant=Passthrough  PCopyVariant=Disabled  TRVariant=Disabled  FdbkBlocksVariant=Forward  IdealPFdbkVariant=Disabled  SatFdbkVariant=Disabled  DerivativeFilterVariant=ContFilter  NVariant=InternalParameters  NCopyVariant=Disabled  FilterICVariant=InternalICsFilter  IntegratorICVariant=InternalICs  ExternalResetVariant=Disabled  TRSumVariant=Passthrough  SumFdbkVariant=Disabled  SumVariant=Sum_PID  TsampFilterVariant=InternalTs  TsampNgainVariant=Passthrough  TsampIntegralVariant=Passthrough  ExternalSaturationOutDataTypeStr=Inherit: Same as second input
  Sum4 : Sum  Inputs=|+-
  Sum5 : Sum  Inputs=|+-
  Torque Controller : pid_lib/PID Controller  Controller=PID  Form=Parallel  TimeDomain=Continuous-time  UseExternalTs=off  SampleTime=0.01  IntegratorMethod=Forward Euler  FilterMethod=Forward Euler  ControllerParametersSource=internal  P=2.50374683332827e-05  I=0.022215359014968  D=0  UseFilter=on  N=100  TunerSelectOption=Transfer Function Based (PID Tuner App)  InitialConditionSource=internal  InitialConditionForIntegrator=0  InitialConditionForFilter=0  DifferentiatorICPrevScaledInput=0  ExternalReset=none  TrackingMode=off  Kt=1  LimitOutput=off  SatLimitsSource=internal  UpperSaturationLimit=inf  LowerSaturationLimit=-inf  LinearizeAsGain=on  AntiWindupMode=none  Kb=1  POutMin=[]  POutMax=[]  IOutMin=[]  IOutMax=[]  DOutMin=[]  DOutMax=[]  NOutMin=[]  NOutMax=[]  SumOutMin=[]  SumOutMax=[]  SaturationOutMin=[]  SaturationOutMax=[]  PParamMin=[]  PParamMax=[]  IParamMin=[]  IParamMax=[]  DParamMin=[]  DParamMax=[]  NParamMin=[]  NParamMax=[]  KbParamMin=[]  KbParamMax=[]  KtParamMin=[]  KtParamMax=[]  KbOutMin=[]  KbOutMax=[]  KtOutMin=[]  KtOutMax=[]  IntegratorOutMin=[]  IntegratorOutMax=[]  FilterOutMin=[]  FilterOutMax=[]  SumI1OutMin=[]  SumI1OutMax=[]  SumI2OutMin=[]  SumI2OutMax=[]  SumI3OutMin=[]  SumI3OutMax=[]  SumI4OutMin=[]  SumI4OutMax=[]  SumDOutMin=[]  SumDOutMax=[]  DifferentiatorOutMin=[]  DifferentiatorOutMax=[]  FilterDiffOutCoefMin=[]  FilterDiffOutCoefMax=[]  ReciprocalOutMin=[]  ReciprocalOutMax=[]  SumDenOutMin=[]  SumDenOutMax=[]  SumNumOutMin=[]  SumNumOutMax=[]  DivideOutMin=[]  DivideOutMax=[]  UdiffTsProdOutMin=[]  UdiffTsProdOutMax=[]  NTsProdOutMin=[]  NTsProdOutMax=[]  UintegralTsProdOutMin=[]  UintegralTsProdOutMax=[]  UngainTsProdOutMin=[]  UngainTsProdOutMax=[]  IntegratorContinuousStateAttributes=''  IntegratorStateMustResolveToSignalObject=off  IntegratorRTWStateStorageClass=Auto  FilterContinuousStateAttributes=''  FilterStateMustResolveToSignalObject=off  FilterRTWStateStorageClass=Auto  ParallelPVariant=InternalParameters  IdealPVariant=Disabled  IVariant=InternalParameters  DVariant=InternalParameters  IntegratorVariant=Continuous  SatVariant=Disabled  AWVariant=Passthrough  PCopyVariant=Disabled  TRVariant=Disabled  FdbkBlocksVariant=Forward  IdealPFdbkVariant=Disabled  SatFdbkVariant=Disabled  DerivativeFilterVariant=ContFilter  NVariant=InternalParameters  NCopyVariant=Disabled  FilterICVariant=InternalICsFilter  IntegratorICVariant=InternalICs  ExternalResetVariant=Disabled  TRSumVariant=Passthrough  SumFdbkVariant=Disabled  SumVariant=Sum_PID  TsampFilterVariant=InternalTs  TsampNgainVariant=Passthrough  TsampIntegralVariant=Passthrough  ExternalSaturationOutDataTypeStr=Inherit: Same as second input
  V limit : Saturate  UpperLimit=20  LowerLimit=-20
  w limit : Saturate  UpperLimit=RW_wmax  LowerLimit=-RW_wmax
  RW1_H : Outport  VectorParamsAs1DForOutWhenUnconnected=off
  RW1_w : Outport  Port=2  VectorParamsAs1DForOutWhenUnconnected=off
  RW1_Hdot : Outport  Port=3  VectorParamsAs1DForOutWhenUnconnected=off
  wires:
  Integrator/1 -> Gain2/1
  RW1_Hdot_des/1 -> Integrator/1
  Mux1/1 -> "Scope Desired and controlled RW-angular speed "/1
  Sum5/1 -> Speed Controller1/1  "M-error"
  RW - DC Motor Model/3(RW_Hrw_dot) -> RW1_Hdot/1, Sum4/2
  Torque Controller/1 -> V limit/1
  Speed Controller1/1 -> w limit/1
  Gain2/1 -> Mux1/1, Sum5/1
  RW - DC Motor Model/2(RW_w) -> RW1_w/1, Sum5/2, Mux1/2
  Sum4/1 -> Torque Controller/1
  w limit/1 -> Sum4/1
  V limit/1 -> RW - DC Motor Model/1(V-rw)  "V-rw"
  RW - DC Motor Model/1(RW_Hrw) -> RW1_H/1

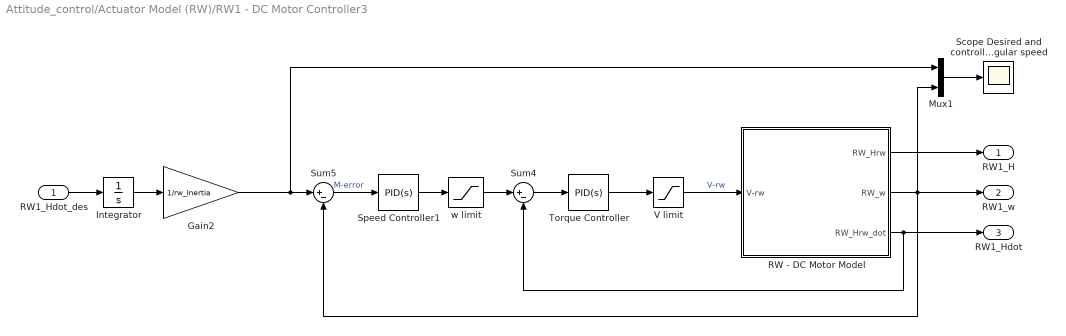
== system Attitude_control/Actuator Model (RW)/RW1 - DC Motor Controller3 ==
  RW1_Hdot_des : Inport
  Gain2 : Gain  Gain=1/rw_Inertia
  Integrator : Integrator
  Mux1 : Mux  Inputs=2
  RW - DC Motor Model : Subsystem
  "Scope Desired and controlled RW-angular speed " : Scope
  Speed Controller1 : pid_lib/PID Controller  Controller=PID  Form=Parallel  TimeDomain=Continuous-time  UseExternalTs=off  SampleTime=0.01  IntegratorMethod=Forward Euler  FilterMethod=Forward Euler  ControllerParametersSource=internal  P=9.56052273582853  I=13.4366327144231  D=1.16248121318414  UseFilter=on  N=2668.95305381072  TunerSelectOption=Transfer Function Based (PID Tuner App)  InitialConditionSource=internal  InitialConditionForIntegrator=0  InitialConditionForFilter=0  DifferentiatorICPrevScaledInput=0  ExternalReset=none  TrackingMode=off  Kt=1  LimitOutput=off  SatLimitsSource=internal  UpperSaturationLimit=inf  LowerSaturationLimit=-inf  LinearizeAsGain=on  AntiWindupMode=none  Kb=1  POutMin=[]  POutMax=[]  IOutMin=[]  IOutMax=[]  DOutMin=[]  DOutMax=[]  NOutMin=[]  NOutMax=[]  SumOutMin=[]  SumOutMax=[]  SaturationOutMin=[]  SaturationOutMax=[]  PParamMin=[]  PParamMax=[]  IParamMin=[]  IParamMax=[]  DParamMin=[]  DParamMax=[]  NParamMin=[]  NParamMax=[]  KbParamMin=[]  KbParamMax=[]  KtParamMin=[]  KtParamMax=[]  KbOutMin=[]  KbOutMax=[]  KtOutMin=[]  KtOutMax=[]  IntegratorOutMin=[]  IntegratorOutMax=[]  FilterOutMin=[]  FilterOutMax=[]  SumI1OutMin=[]  SumI1OutMax=[]  SumI2OutMin=[]  SumI2OutMax=[]  SumI3OutMin=[]  SumI3OutMax=[]  SumI4OutMin=[]  SumI4OutMax=[]  SumDOutMin=[]  SumDOutMax=[]  DifferentiatorOutMin=[]  DifferentiatorOutMax=[]  FilterDiffOutCoefMin=[]  FilterDiffOutCoefMax=[]  ReciprocalOutMin=[]  ReciprocalOutMax=[]  SumDenOutMin=[]  SumDenOutMax=[]  SumNumOutMin=[]  SumNumOutMax=[]  DivideOutMin=[]  DivideOutMax=[]  UdiffTsProdOutMin=[]  UdiffTsProdOutMax=[]  NTsProdOutMin=[]  NTsProdOutMax=[]  UintegralTsProdOutMin=[]  UintegralTsProdOutMax=[]  UngainTsProdOutMin=[]  UngainTsProdOutMax=[]  IntegratorContinuousStateAttributes=''  IntegratorStateMustResolveToSignalObject=off  IntegratorRTWStateStorageClass=Auto  FilterContinuousStateAttributes=''  FilterStateMustResolveToSignalObject=off  FilterRTWStateStorageClass=Auto  ParallelPVariant=InternalParameters  IdealPVariant=Disabled  IVariant=InternalParameters  DVariant=InternalParameters  IntegratorVariant=Continuous  SatVariant=Disabled  AWVariant=Passthrough  PCopyVariant=Disabled  TRVariant=Disabled  FdbkBlocksVariant=Forward  IdealPFdbkVariant=Disabled  SatFdbkVariant=Disabled  DerivativeFilterVariant=ContFilter  NVariant=InternalParameters  NCopyVariant=Disabled  FilterICVariant=InternalICsFilter  IntegratorICVariant=InternalICs  ExternalResetVariant=Disabled  TRSumVariant=Passthrough  SumFdbkVariant=Disabled  SumVariant=Sum_PID  TsampFilterVariant=InternalTs  TsampNgainVariant=Passthrough  TsampIntegralVariant=Passthrough  ExternalSaturationOutDataTypeStr=Inherit: Same as second input
  Sum4 : Sum  Inputs=|+-
  Sum5 : Sum  Inputs=|+-
  Torque Controller : pid_lib/PID Controller  Controller=PID  Form=Parallel  TimeDomain=Continuous-time  UseExternalTs=off  SampleTime=0.01  IntegratorMethod=Forward Euler  FilterMethod=Forward Euler  ControllerParametersSource=internal  P=2.50374683332827e-05  I=0.022215359014968  D=0  UseFilter=on  N=100  TunerSelectOption=Transfer Function Based (PID Tuner App)  InitialConditionSource=internal  InitialConditionForIntegrator=0  InitialConditionForFilter=0  DifferentiatorICPrevScaledInput=0  ExternalReset=none  TrackingMode=off  Kt=1  LimitOutput=off  SatLimitsSource=internal  UpperSaturationLimit=inf  LowerSaturationLimit=-inf  LinearizeAsGain=on  AntiWindupMode=none  Kb=1  POutMin=[]  POutMax=[]  IOutMin=[]  IOutMax=[]  DOutMin=[]  DOutMax=[]  NOutMin=[]  NOutMax=[]  SumOutMin=[]  SumOutMax=[]  SaturationOutMin=[]  SaturationOutMax=[]  PParamMin=[]  PParamMax=[]  IParamMin=[]  IParamMax=[]  DParamMin=[]  DParamMax=[]  NParamMin=[]  NParamMax=[]  KbParamMin=[]  KbParamMax=[]  KtParamMin=[]  KtParamMax=[]  KbOutMin=[]  KbOutMax=[]  KtOutMin=[]  KtOutMax=[]  IntegratorOutMin=[]  IntegratorOutMax=[]  FilterOutMin=[]  FilterOutMax=[]  SumI1OutMin=[]  SumI1OutMax=[]  SumI2OutMin=[]  SumI2OutMax=[]  SumI3OutMin=[]  SumI3OutMax=[]  SumI4OutMin=[]  SumI4OutMax=[]  SumDOutMin=[]  SumDOutMax=[]  DifferentiatorOutMin=[]  DifferentiatorOutMax=[]  FilterDiffOutCoefMin=[]  FilterDiffOutCoefMax=[]  ReciprocalOutMin=[]  ReciprocalOutMax=[]  SumDenOutMin=[]  SumDenOutMax=[]  SumNumOutMin=[]  SumNumOutMax=[]  DivideOutMin=[]  DivideOutMax=[]  UdiffTsProdOutMin=[]  UdiffTsProdOutMax=[]  NTsProdOutMin=[]  NTsProdOutMax=[]  UintegralTsProdOutMin=[]  UintegralTsProdOutMax=[]  UngainTsProdOutMin=[]  UngainTsProdOutMax=[]  IntegratorContinuousStateAttributes=''  IntegratorStateMustResolveToSignalObject=off  IntegratorRTWStateStorageClass=Auto  FilterContinuousStateAttributes=''  FilterStateMustResolveToSignalObject=off  FilterRTWStateStorageClass=Auto  ParallelPVariant=InternalParameters  IdealPVariant=Disabled  IVariant=InternalParameters  DVariant=InternalParameters  IntegratorVariant=Continuous  SatVariant=Disabled  AWVariant=Passthrough  PCopyVariant=Disabled  TRVariant=Disabled  FdbkBlocksVariant=Forward  IdealPFdbkVariant=Disabled  SatFdbkVariant=Disabled  DerivativeFilterVariant=ContFilter  NVariant=InternalParameters  NCopyVariant=Disabled  FilterICVariant=InternalICsFilter  IntegratorICVariant=InternalICs  ExternalResetVariant=Disabled  TRSumVariant=Passthrough  SumFdbkVariant=Disabled  SumVariant=Sum_PID  TsampFilterVariant=InternalTs  TsampNgainVariant=Passthrough  TsampIntegralVariant=Passthrough  ExternalSaturationOutDataTypeStr=Inherit: Same as second input
  V limit : Saturate  UpperLimit=20  LowerLimit=-20
  w limit : Saturate  UpperLimit=RW_wmax  LowerLimit=-RW_wmax
  RW1_H : Outport  VectorParamsAs1DForOutWhenUnconnected=off
  RW1_w : Outport  Port=2  VectorParamsAs1DForOutWhenUnconnected=off
  RW1_Hdot : Outport  Port=3  VectorParamsAs1DForOutWhenUnconnected=off
  wires:
  Integrator/1 -> Gain2/1
  RW1_Hdot_des/1 -> Integrator/1
  Mux1/1 -> "Scope Desired and controlled RW-angular speed "/1
  Sum5/1 -> Speed Controller1/1  "M-error"
  RW - DC Motor Model/3(RW_Hrw_dot) -> RW1_Hdot/1, Sum4/2
  Torque Controller/1 -> V limit/1
  Speed Controller1/1 -> w limit/1
  Gain2/1 -> Mux1/1, Sum5/1
  RW - DC Motor Model/2(RW_w) -> RW1_w/1, Sum5/2, Mux1/2
  Sum4/1 -> Torque Controller/1
  w limit/1 -> Sum4/1
  V limit/1 -> RW - DC Motor Model/1(V-rw)  "V-rw"
  RW - DC Motor Model/1(RW_Hrw) -> RW1_H/1

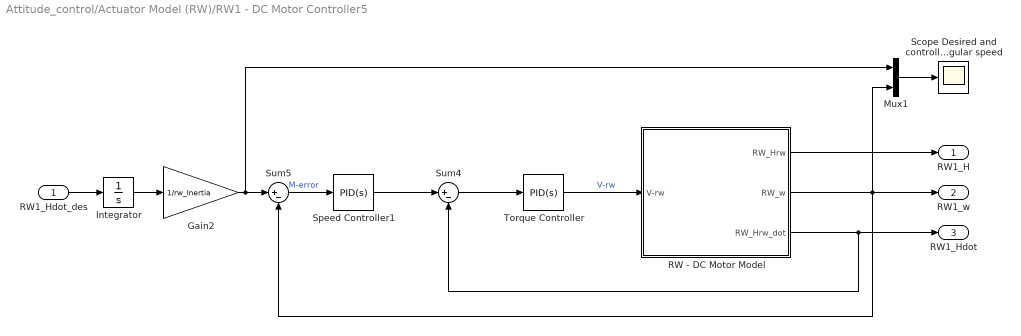
== system Attitude_control/Actuator Model (RW)/RW1 - DC Motor Controller5 ==
  RW1_Hdot_des : Inport
  Gain2 : Gain  Gain=1/rw_Inertia
  Integrator : Integrator
  Mux1 : Mux  Inputs=2
  RW - DC Motor Model : Subsystem
  "Scope Desired and controlled RW-angular speed " : Scope
  Speed Controller1 : pid_lib/PID Controller  Controller=PID  Form=Parallel  TimeDomain=Continuous-time  UseExternalTs=off  SampleTime=0.01  IntegratorMethod=Forward Euler  FilterMethod=Forward Euler  ControllerParametersSource=internal  P=9.56052273582853  I=13.4366327144231  D=1.16248121318414  UseFilter=on  N=2668.95305381072  TunerSelectOption=Transfer Function Based (PID Tuner App)  InitialConditionSource=internal  InitialConditionForIntegrator=0  InitialConditionForFilter=0  DifferentiatorICPrevScaledInput=0  ExternalReset=none  TrackingMode=off  Kt=1  LimitOutput=off  SatLimitsSource=internal  UpperSaturationLimit=inf  LowerSaturationLimit=-inf  LinearizeAsGain=on  AntiWindupMode=none  Kb=1  POutMin=[]  POutMax=[]  IOutMin=[]  IOutMax=[]  DOutMin=[]  DOutMax=[]  NOutMin=[]  NOutMax=[]  SumOutMin=[]  SumOutMax=[]  SaturationOutMin=[]  SaturationOutMax=[]  PParamMin=[]  PParamMax=[]  IParamMin=[]  IParamMax=[]  DParamMin=[]  DParamMax=[]  NParamMin=[]  NParamMax=[]  KbParamMin=[]  KbParamMax=[]  KtParamMin=[]  KtParamMax=[]  KbOutMin=[]  KbOutMax=[]  KtOutMin=[]  KtOutMax=[]  IntegratorOutMin=[]  IntegratorOutMax=[]  FilterOutMin=[]  FilterOutMax=[]  SumI1OutMin=[]  SumI1OutMax=[]  SumI2OutMin=[]  SumI2OutMax=[]  SumI3OutMin=[]  SumI3OutMax=[]  SumI4OutMin=[]  SumI4OutMax=[]  SumDOutMin=[]  SumDOutMax=[]  DifferentiatorOutMin=[]  DifferentiatorOutMax=[]  FilterDiffOutCoefMin=[]  FilterDiffOutCoefMax=[]  ReciprocalOutMin=[]  ReciprocalOutMax=[]  SumDenOutMin=[]  SumDenOutMax=[]  SumNumOutMin=[]  SumNumOutMax=[]  DivideOutMin=[]  DivideOutMax=[]  UdiffTsProdOutMin=[]  UdiffTsProdOutMax=[]  NTsProdOutMin=[]  NTsProdOutMax=[]  UintegralTsProdOutMin=[]  UintegralTsProdOutMax=[]  UngainTsProdOutMin=[]  UngainTsProdOutMax=[]  IntegratorContinuousStateAttributes=''  IntegratorStateMustResolveToSignalObject=off  IntegratorRTWStateStorageClass=Auto  FilterContinuousStateAttributes=''  FilterStateMustResolveToSignalObject=off  FilterRTWStateStorageClass=Auto  ParallelPVariant=InternalParameters  IdealPVariant=Disabled  IVariant=InternalParameters  DVariant=InternalParameters  IntegratorVariant=Continuous  SatVariant=Disabled  AWVariant=Passthrough  PCopyVariant=Disabled  TRVariant=Disabled  FdbkBlocksVariant=Forward  IdealPFdbkVariant=Disabled  SatFdbkVariant=Disabled  DerivativeFilterVariant=ContFilter  NVariant=InternalParameters  NCopyVariant=Disabled  FilterICVariant=InternalICsFilter  IntegratorICVariant=InternalICs  ExternalResetVariant=Disabled  TRSumVariant=Passthrough  SumFdbkVariant=Disabled  SumVariant=Sum_PID  TsampFilterVariant=InternalTs  TsampNgainVariant=Passthrough  TsampIntegralVariant=Passthrough  ExternalSaturationOutDataTypeStr=Inherit: Same as second input
  Sum4 : Sum  Inputs=|+-
  Sum5 : Sum  Inputs=|+-
  Torque Controller : pid_lib/PID Controller  Controller=PID  Form=Parallel  TimeDomain=Continuous-time  UseExternalTs=off  SampleTime=0.01  IntegratorMethod=Forward Euler  FilterMethod=Forward Euler  ControllerParametersSource=internal  P=2.50374683332827e-05  I=0.022215359014968  D=0  UseFilter=on  N=100  TunerSelectOption=Transfer Function Based (PID Tuner App)  InitialConditionSource=internal  InitialConditionForIntegrator=0  InitialConditionForFilter=0  DifferentiatorICPrevScaledInput=0  ExternalReset=none  TrackingMode=off  Kt=1  LimitOutput=off  SatLimitsSource=internal  UpperSaturationLimit=inf  LowerSaturationLimit=-inf  LinearizeAsGain=on  AntiWindupMode=none  Kb=1  POutMin=[]  POutMax=[]  IOutMin=[]  IOutMax=[]  DOutMin=[]  DOutMax=[]  NOutMin=[]  NOutMax=[]  SumOutMin=[]  SumOutMax=[]  SaturationOutMin=[]  SaturationOutMax=[]  PParamMin=[]  PParamMax=[]  IParamMin=[]  IParamMax=[]  DParamMin=[]  DParamMax=[]  NParamMin=[]  NParamMax=[]  KbParamMin=[]  KbParamMax=[]  KtParamMin=[]  KtParamMax=[]  KbOutMin=[]  KbOutMax=[]  KtOutMin=[]  KtOutMax=[]  IntegratorOutMin=[]  IntegratorOutMax=[]  FilterOutMin=[]  FilterOutMax=[]  SumI1OutMin=[]  SumI1OutMax=[]  SumI2OutMin=[]  SumI2OutMax=[]  SumI3OutMin=[]  SumI3OutMax=[]  SumI4OutMin=[]  SumI4OutMax=[]  SumDOutMin=[]  SumDOutMax=[]  DifferentiatorOutMin=[]  DifferentiatorOutMax=[]  FilterDiffOutCoefMin=[]  FilterDiffOutCoefMax=[]  ReciprocalOutMin=[]  ReciprocalOutMax=[]  SumDenOutMin=[]  SumDenOutMax=[]  SumNumOutMin=[]  SumNumOutMax=[]  DivideOutMin=[]  DivideOutMax=[]  UdiffTsProdOutMin=[]  UdiffTsProdOutMax=[]  NTsProdOutMin=[]  NTsProdOutMax=[]  UintegralTsProdOutMin=[]  UintegralTsProdOutMax=[]  UngainTsProdOutMin=[]  UngainTsProdOutMax=[]  IntegratorContinuousStateAttributes=''  IntegratorStateMustResolveToSignalObject=off  IntegratorRTWStateStorageClass=Auto  FilterContinuousStateAttributes=''  FilterStateMustResolveToSignalObject=off  FilterRTWStateStorageClass=Auto  ParallelPVariant=InternalParameters  IdealPVariant=Disabled  IVariant=InternalParameters  DVariant=InternalParameters  IntegratorVariant=Continuous  SatVariant=Disabled  AWVariant=Passthrough  PCopyVariant=Disabled  TRVariant=Disabled  FdbkBlocksVariant=Forward  IdealPFdbkVariant=Disabled  SatFdbkVariant=Disabled  DerivativeFilterVariant=ContFilter  NVariant=InternalParameters  NCopyVariant=Disabled  FilterICVariant=InternalICsFilter  IntegratorICVariant=InternalICs  ExternalResetVariant=Disabled  TRSumVariant=Passthrough  SumFdbkVariant=Disabled  SumVariant=Sum_PID  TsampFilterVariant=InternalTs  TsampNgainVariant=Passthrough  TsampIntegralVariant=Passthrough  ExternalSaturationOutDataTypeStr=Inherit: Same as second input
  RW1_H : Outport  VectorParamsAs1DForOutWhenUnconnected=off
  RW1_w : Outport  Port=2  VectorParamsAs1DForOutWhenUnconnected=off
  RW1_Hdot : Outport  Port=3  VectorParamsAs1DForOutWhenUnconnected=off
  wires:
  Integrator/1 -> Gain2/1
  RW1_Hdot_des/1 -> Integrator/1
  RW - DC Motor Model/1(RW_Hrw) -> RW1_H/1
  Sum4/1 -> Torque Controller/1
  RW - DC Motor Model/2(RW_w) -> RW1_w/1, Sum5/2, Mux1/2
  Speed Controller1/1 -> Sum4/1
  Sum5/1 -> Speed Controller1/1  "M-error"
  Torque Controller/1 -> RW - DC Motor Model/1(V-rw)  "V-rw"
  Mux1/1 -> "Scope Desired and controlled RW-angular speed "/1
  RW - DC Motor Model/3(RW_Hrw_dot) -> RW1_Hdot/1, Sum4/2
  Gain2/1 -> Mux1/1, Sum5/1

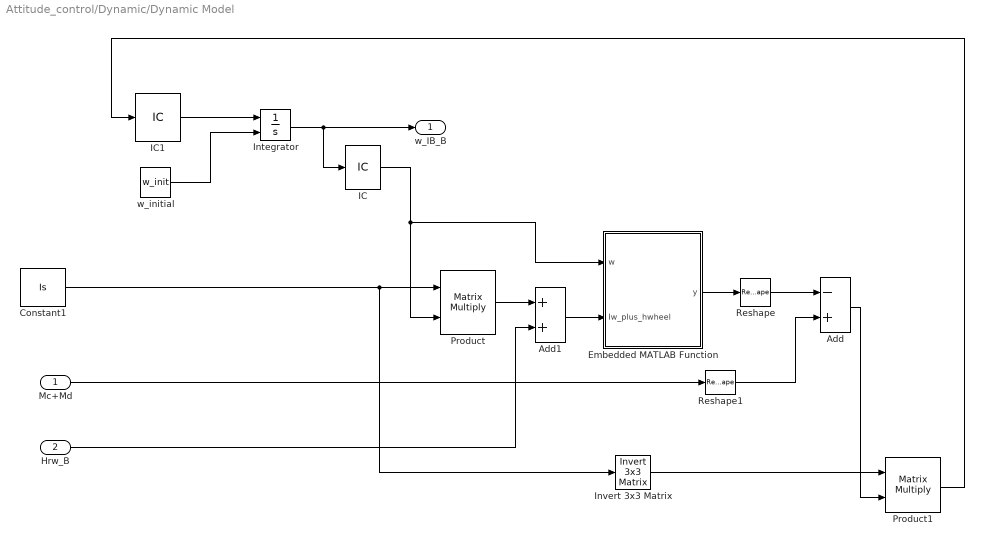
== system Attitude_control/Dynamic/Dynamic Model ==
  Mc+Md : Inport
  "Hrw_B " : Inport  Port=2
  Add : Sum  Inputs=-+
  Add1 : Sum
  Constant1 : Constant  Value=Is
  Embedded MATLAB Function : MATLAB Function  TreatAsAtomicUnit=on
  IC : InitialCondition  Value=w_init
  IC1 : InitialCondition  Value=w_dot_init
  Integrator : Integrator  InitialConditionSource=external  InitialCondition=[0;0;0]
  Invert 3x3 Matrix : aerolibutil/Invert  3x3 Matrix
  Product : Product  Multiplication=Matrix(*)  RndMeth=Zero
  Product1 : Product  Multiplication=Matrix(*)  RndMeth=Zero
  Reshape : Reshape  OutputDimensionality=Column vector (2-D)
  Reshape1 : Reshape  OutputDimensionality=Column vector (2-D)
  w_initial : Constant  Value=w_init  VectorParams1D=off  SampleTime=-1
  w_IB_B : Outport  VectorParamsAs1DForOutWhenUnconnected=off
  wires:
  Constant1/1 -> Invert 3x3 Matrix/1, Product/1
  IC/1 -> Product/2, Embedded MATLAB Function/1(w)
  Mc+Md/1 -> Reshape1/1
  Invert 3x3 Matrix/1 -> Product1/1
  Integrator/1 -> w_IB_B/1, IC/1
  Product1/1 -> IC1/1
  Embedded MATLAB Function/1(y) -> Reshape/1
  w_initial/1 -> Integrator/2
  Add/1 -> Product1/2
  IC1/1 -> Integrator/1
  Reshape/1 -> Add/1
  Reshape1/1 -> Add/2
  Product/1 -> Add1/1
  Add1/1 -> Embedded MATLAB Function/2(Iw_plus_hwheel)
  "Hrw_B "/1 -> Add1/2
